simulink model "c00026M_harness"  (R2018a)
settings: Solver=ode3  StartTime=0.0  StopTime=10.0  RelTol=1e-3  EnableMultiTasking=on
undefined symbols (not defined in the file): b, DiscIntNeverNeededParam, J, K, L, PosMinimaW4, R, sigbuilder_block
(part 35 of 40)

== stateflow chart c00026M_harness/M063/Cyber/WL/Chart ==
  state Bajand_hasta_abajo
    entry: W = -1;
  state Bajando
    entry: W = -1;
  state Idle
    entry:W = 0;
  state Subiendo_hasta_arriba
    entry: W = 1;
  state Subiendo
    entry: W = 1;
  Subiendo -> Bajand_hasta_abajo [order 4] : [UI==4]
  Bajand_hasta_abajo -> Bajando [order 2] : [UI==3]
  Subiendo -> Bajando [order 3] : [UI==3]
  Bajando -> Bajand_hasta_abajo [order 2] : [UI==4]
  Idle -> Bajando [order 3] : [UI==3&&S>0]
  Subiendo_hasta_arriba -> Bajand_hasta_abajo [order 3] : [UI==4]
  Idle -> Bajand_hasta_abajo [order 4] : [UI==4&&S>0]
  Bajando -> Subiendo [order 3] : [UI==1]
  Subiendo_hasta_arriba -> Bajando [order 4] : [UI==3]
  Bajand_hasta_abajo -> Subiendo [order 4] : [UI==1]
  Bajand_hasta_abajo -> Idle [order 1] : [S<=0]
  Bajand_hasta_abajo -> Subiendo_hasta_arriba [order 3] : [UI==2]
  Bajando -> Idle [order 1] : [S<=0||UI==0]
  Bajando -> Subiendo_hasta_arriba [order 4] : [UI==2]
  (default) -> Idle
  Idle -> Subiendo_hasta_arriba [order 2] : [UI>2&&S<5]
  Idle -> Subiendo [order 1] : [UI == 1&&S<5]
  Subiendo -> Idle [order 1] : [S>=5||UI==0]
  Subiendo_hasta_arriba -> Idle [order 1] : [S >=5]
  Subiendo_hasta_arriba -> Subiendo [order 2] : [UI ==1]
  Subiendo -> Subiendo_hasta_arriba [order 2] : [UI==2]
  data: S input; UI input; W output double

== stateflow chart c00026M_harness/M063/Cyber/WL1/Chart1 ==
  state Bajand_hasta_abajo
    entry: W = -1;
  state Bajando
    entry: W = -1;
  state Idle
    entry:W = 0;
  state Subiendo_hasta_arriba
    entry: W = 1;
  state Subiendo
    entry: W = 1;
  Subiendo -> Bajand_hasta_abajo [order 4] : [UI==4]
  Bajand_hasta_abajo -> Bajando [order 2] : [UI==3]
  Subiendo -> Bajando [order 3] : [UI==3]
  Bajando -> Bajand_hasta_abajo [order 2] : [UI==4]
  Idle -> Bajando [order 3] : [UI==3&&S>0]
  Subiendo_hasta_arriba -> Bajand_hasta_abajo [order 3] : [UI==4]
  Idle -> Bajand_hasta_abajo [order 4] : [UI==4&&S>0]
  Bajando -> Subiendo [order 3] : [UI==1]
  Subiendo_hasta_arriba -> Bajando [order 4] : [UI==3]
  Bajand_hasta_abajo -> Subiendo [order 4] : [UI==1]
  Bajand_hasta_abajo -> Idle [order 1] : [S<=0]
  Bajand_hasta_abajo -> Subiendo_hasta_arriba [order 3] : [UI==2]
  Bajando -> Idle [order 1] : [S<=0||UI==0]
  Bajando -> Subiendo_hasta_arriba [order 4] : [UI==2]
  (default) -> Idle
  Idle -> Subiendo_hasta_arriba [order 2] : [UI==2&&S<5]
  Idle -> Subiendo [order 1] : [UI == 1&&S<5]
  Subiendo -> Idle [order 1] : [S>=5||UI==0]
  Subiendo_hasta_arriba -> Idle [order 1] : [S >=5]
  Subiendo_hasta_arriba -> Subiendo [order 2] : [UI ==1]
  Subiendo -> Subiendo_hasta_arriba [order 2] : [UI==2]
  data: S input; UI input; W output double

== stateflow chart c00026M_harness/M063/Cyber/WL3/Chart2 ==
  state Bajand_hasta_abajo
    entry: W = -1;
  state Bajando
    entry: W = -1;
  state Idle
    entry:W = 0;
  state Subiendo_hasta_arriba
    entry: W = 1;
  state Subiendo
    entry: W = 1;
  Subiendo -> Bajand_hasta_abajo [order 4] : [UI==4]
  Bajand_hasta_abajo -> Bajando [order 2] : [UI==3]
  Subiendo -> Bajando [order 3] : [UI==3]
  Bajando -> Bajand_hasta_abajo [order 2] : [UI==4]
  Idle -> Bajando [order 3] : [UI==3&&S>PosMinW4]
  Subiendo_hasta_arriba -> Bajand_hasta_abajo [order 3] : [UI==4]
  Idle -> Bajand_hasta_abajo [order 4] : [UI==4&&S>PosMinW4]
  Bajando -> Subiendo [order 3] : [UI==1]
  Subiendo_hasta_arriba -> Bajando [order 4] : [UI==3]
  Bajand_hasta_abajo -> Subiendo [order 4] : [UI==1]
  Bajand_hasta_abajo -> Idle [order 1] : [S<=PosMinW4]
  Bajand_hasta_abajo -> Subiendo_hasta_arriba [order 3] : [UI==2]
  Bajando -> Idle [order 1] : [S<=PosMinW4||UI==0]
  Bajando -> Subiendo_hasta_arriba [order 4] : [UI==2]
  (default) -> Idle
  Idle -> Subiendo_hasta_arriba [order 2] : [UI==2&&S<5]
  Idle -> Subiendo [order 1] : [UI == 1&&S<5]
  Subiendo -> Idle [order 1] : [S>=5||UI==0]
  Subiendo_hasta_arriba -> Idle [order 1] : [S >=5]
  Subiendo_hasta_arriba -> Subiendo [order 2] : [UI ==1]
  Subiendo -> Subiendo_hasta_arriba [order 2] : [UI==2]
  data: S input; UI input; W output double; PosMinW4 input

== stateflow chart c00026M_harness/M064/Cyber/WL/Chart ==
  state Bajand_hasta_abajo
    entry: W = -1;
  state Bajando
    entry: W = -1;
  state Idle
    entry:W = 0;
  state Subiendo_hasta_arriba
    entry: W = 1;
  state Subiendo
    entry: W = 1;
  Subiendo -> Bajand_hasta_abajo [order 4] : [UI==4]
  Bajand_hasta_abajo -> Bajando [order 2] : [UI==3]
  Subiendo -> Bajando [order 3] : [UI==3]
  Bajando -> Bajand_hasta_abajo [order 2] : [UI==4]
  Idle -> Bajando [order 3] : [UI==3&&S>0]
  Subiendo_hasta_arriba -> Bajand_hasta_abajo [order 3] : [UI==4]
  Idle -> Bajand_hasta_abajo [order 4] : [UI==4&&S>0]
  Bajando -> Subiendo [order 3] : [UI==1]
  Subiendo_hasta_arriba -> Bajando [order 4] : [UI==3]
  Bajand_hasta_abajo -> Subiendo [order 4] : [UI==1]
  Bajand_hasta_abajo -> Idle [order 1] : [S<=0]
  Bajand_hasta_abajo -> Subiendo_hasta_arriba [order 3] : [UI==2]
  Bajando -> Idle [order 1] : [S<=0||UI==0]
  Bajando -> Subiendo_hasta_arriba [order 4] : [UI==2]
  (default) -> Idle
  Idle -> Subiendo_hasta_arriba [order 2] : [UI==2&&S<5]
  Idle -> Subiendo [order 1] : [UI == 1&&S<5]
  Subiendo -> Idle [order 1] : [S>=5||UI==0]
  Subiendo_hasta_arriba -> Idle [order 1] : [S >=5]
  Subiendo_hasta_arriba -> Subiendo [order 2] : [UI ==1]
  Subiendo -> Subiendo_hasta_arriba [order 2] : [UI==2]
  data: S input; UI input; W output double

== stateflow chart c00026M_harness/M064/Cyber/WL1/Chart1 ==
  state Bajand_hasta_abajo
    entry: W = -1;
  state Bajando
    entry: W = -1;
  state Idle
    entry:W = 0;
  state Subiendo_hasta_arriba
    entry: W = 1;
  state Subiendo
    entry: W = 1;
  Subiendo -> Bajand_hasta_abajo [order 4] : [UI==4]
  Bajand_hasta_abajo -> Bajando [order 2] : [UI==3]
  Subiendo -> Bajando [order 3] : [UI==3]
  Bajando -> Bajand_hasta_abajo [order 2] : [UI==4]
  Idle -> Bajando [order 3] : [UI==3&&S>0]
  Subiendo_hasta_arriba -> Bajand_hasta_abajo [order 3] : [UI==4]
  Idle -> Bajand_hasta_abajo [order 4] : [UI==4&&S>0]
  Bajando -> Subiendo [order 3] : [UI==1]
  Subiendo_hasta_arriba -> Bajando [order 4] : [UI==3]
  Bajand_hasta_abajo -> Subiendo [order 4] : [UI==1]
  Bajand_hasta_abajo -> Idle [order 1] : [S<=0]
  Bajand_hasta_abajo -> Subiendo_hasta_arriba [order 3] : [UI==2]
  Bajando -> Idle [order 1] : [S<=0||UI==0]
  Bajando -> Subiendo_hasta_arriba [order 4] : [UI==2]
  (default) -> Idle
  Idle -> Subiendo_hasta_arriba [order 2] : [UI>2&&S<5]
  Idle -> Subiendo [order 1] : [UI == 1&&S<5]
  Subiendo -> Idle [order 1] : [S>=5||UI==0]
  Subiendo_hasta_arriba -> Idle [order 1] : [S >=5]
  Subiendo_hasta_arriba -> Subiendo [order 2] : [UI ==1]
  Subiendo -> Subiendo_hasta_arriba [order 2] : [UI==2]
  data: S input; UI input; W output double

== stateflow chart c00026M_harness/M064/Cyber/WL3/Chart2 ==
  state Bajand_hasta_abajo
    entry: W = -1;
  state Bajando
    entry: W = -1;
  state Idle
    entry:W = 0;
  state Subiendo_hasta_arriba
    entry: W = 1;
  state Subiendo
    entry: W = 1;
  Subiendo -> Bajand_hasta_abajo [order 4] : [UI==4]
  Bajand_hasta_abajo -> Bajando [order 2] : [UI==3]
  Subiendo -> Bajando [order 3] : [UI==3]
  Bajando -> Bajand_hasta_abajo [order 2] : [UI==4]
  Idle -> Bajando [order 3] : [UI==3&&S>PosMinW4]
  Subiendo_hasta_arriba -> Bajand_hasta_abajo [order 3] : [UI==4]
  Idle -> Bajand_hasta_abajo [order 4] : [UI==4&&S>PosMinW4]
  Bajando -> Subiendo [order 3] : [UI==1]
  Subiendo_hasta_arriba -> Bajando [order 4] : [UI==3]
  Bajand_hasta_abajo -> Subiendo [order 4] : [UI==1]
  Bajand_hasta_abajo -> Idle [order 1] : [S<=PosMinW4]
  Bajand_hasta_abajo -> Subiendo_hasta_arriba [order 3] : [UI==2]
  Bajando -> Idle [order 1] : [S<=PosMinW4||UI==0]
  Bajando -> Subiendo_hasta_arriba [order 4] : [UI==2]
  (default) -> Idle
  Idle -> Subiendo_hasta_arriba [order 2] : [UI==2&&S<5]
  Idle -> Subiendo [order 1] : [UI == 1&&S<5]
  Subiendo -> Idle [order 1] : [S>=5||UI==0]
  Subiendo_hasta_arriba -> Idle [order 1] : [S >=5]
  Subiendo_hasta_arriba -> Subiendo [order 2] : [UI ==1]
  Subiendo -> Subiendo_hasta_arriba [order 2] : [UI==2]
  data: S input; UI input; W output double; PosMinW4 input

== stateflow chart c00026M_harness/M066/Cyber/WL/Chart ==
  state Bajand_hasta_abajo
    entry: W = -1;
  state Bajando
    entry: W = -1;
  state Idle
    entry:W = 0;
  state Subiendo_hasta_arriba
    entry: W = 1;
  state Subiendo
    entry: W = 1;
  Subiendo -> Bajand_hasta_abajo [order 4] : [UI==4]
  Bajand_hasta_abajo -> Bajando [order 2] : [UI==3]
  Subiendo -> Bajando [order 3] : [UI==3]
  Bajando -> Bajand_hasta_abajo [order 2] : [UI==4]
  Idle -> Bajando [order 3] : [UI==3&&S>0]
  Subiendo_hasta_arriba -> Bajand_hasta_abajo [order 3] : [UI==4]
  Idle -> Bajand_hasta_abajo [order 4] : [UI==4&&S>0]
  Bajando -> Subiendo [order 3] : [UI==1]
  Subiendo_hasta_arriba -> Bajando [order 4] : [UI==3]
  Bajand_hasta_abajo -> Subiendo [order 4] : [UI==1]
  Bajand_hasta_abajo -> Idle [order 1] : [S<=0]
  Bajand_hasta_abajo -> Subiendo_hasta_arriba [order 3] : [UI==2]
  Bajando -> Idle [order 1] : [S<=0||UI==0]
  Bajando -> Subiendo_hasta_arriba [order 4] : [UI==2]
  (default) -> Idle
  Idle -> Subiendo_hasta_arriba [order 2] : [UI==2&&S<5]
  Idle -> Subiendo [order 1] : [UI == 1&&S<5]
  Subiendo -> Idle [order 1] : [S>=5||UI==0]
  Subiendo_hasta_arriba -> Idle [order 1] : [S >=5]
  Subiendo_hasta_arriba -> Subiendo [order 2] : [UI ==1]
  Subiendo -> Subiendo_hasta_arriba [order 2] : [UI==2]
  data: S input; UI input; W output double

== stateflow chart c00026M_harness/M066/Cyber/WL1/Chart1 ==
  state Bajand_hasta_abajo
    entry: W = -1;
  state Bajando
    entry: W = -1;
  state Idle
    entry:W = 0;
  state Subiendo_hasta_arriba
    entry: W = 1;
  state Subiendo
    entry: W = 1;
  Subiendo -> Bajand_hasta_abajo [order 4] : [UI==4]
  Bajand_hasta_abajo -> Bajando [order 2] : [UI==3]
  Subiendo -> Bajando [order 3] : [UI==3]
  Bajando -> Bajand_hasta_abajo [order 2] : [UI==4]
  Idle -> Bajando [order 3] : [UI==3&&S>0]
  Subiendo_hasta_arriba -> Bajand_hasta_abajo [order 3] : [UI==4]
  Idle -> Bajand_hasta_abajo [order 4] : [UI==4&&S>0]
  Bajando -> Subiendo [order 3] : [UI==1]
  Subiendo_hasta_arriba -> Bajando [order 4] : [UI==3]
  Bajand_hasta_abajo -> Subiendo [order 4] : [UI==1]
  Bajand_hasta_abajo -> Idle [order 1] : [S<=0]
  Bajand_hasta_abajo -> Subiendo_hasta_arriba [order 3] : [UI==2]
  Bajando -> Idle [order 1] : [S<=0||UI==0]
  Bajando -> Subiendo_hasta_arriba [order 4] : [UI==2]
  (default) -> Idle
  Idle -> Subiendo_hasta_arriba [order 2] : [UI==2&&S<5]
  Idle -> Subiendo [order 1] : [UI == 1&&S<5]
  Subiendo -> Idle [order 1] : [S>=5||UI==0]
  Subiendo_hasta_arriba -> Idle [order 1] : [S >=5]
  Subiendo_hasta_arriba -> Subiendo [order 2] : [UI ==1]
  Subiendo -> Subiendo_hasta_arriba [order 2] : [UI==2]
  data: S input; UI input; W output double

== stateflow chart c00026M_harness/M066/Cyber/WL3/Chart2 ==
  state Bajand_hasta_abajo
    entry: W = -1;
  state Bajando
    entry: W = -1;
  state Idle
    entry:W = 0;
  state Subiendo_hasta_arriba
    entry: W = 1;
  state Subiendo
    entry: W = 1;
  Subiendo -> Bajand_hasta_abajo [order 4] : [UI==4]
  Bajand_hasta_abajo -> Bajando [order 2] : [UI==3]
  Subiendo -> Bajando [order 3] : [UI==3]
  Bajando -> Bajand_hasta_abajo [order 2] : [UI==4]
  Idle -> Bajando [order 3] : [UI==3&&S>PosMinW4]
  Subiendo_hasta_arriba -> Bajand_hasta_abajo [order 3] : [UI==4]
  Idle -> Bajand_hasta_abajo [order 4] : [UI==4&&S>PosMinW4]
  Bajando -> Subiendo [order 3] : [UI==1]
  Subiendo_hasta_arriba -> Bajando [order 4] : [UI==3]
  Bajand_hasta_abajo -> Subiendo [order 4] : [UI==1]
  Bajand_hasta_abajo -> Idle [order 1] : [S<=PosMinW4]
  Bajand_hasta_abajo -> Subiendo_hasta_arriba [order 3] : [UI==2]
  Bajando -> Idle [order 1] : [S<=PosMinW4||UI==0]
  Bajando -> Subiendo_hasta_arriba [order 4] : [UI==2]
  (default) -> Idle
  Idle -> Subiendo_hasta_arriba [order 2] : [UI>2&&S<5]
  Idle -> Subiendo [order 1] : [UI == 1&&S<5]
  Subiendo -> Idle [order 1] : [S>=5||UI==0]
  Subiendo_hasta_arriba -> Idle [order 1] : [S >=5]
  Subiendo_hasta_arriba -> Subiendo [order 2] : [UI ==1]
  Subiendo -> Subiendo_hasta_arriba [order 2] : [UI==2]
  data: S input; UI input; W output double; PosMinW4 input

== stateflow chart c00026M_harness/M067/Cyber/WL/Chart ==
  state Bajand_hasta_abajo
    entry: W = -1;
  state Bajando
    entry: W = -1;
  state Idle
    entry:W = 0;
  state Subiendo_hasta_arriba
    entry: W = 1;
  state Subiendo
    entry: W = 1;
  Subiendo -> Bajand_hasta_abajo [order 4] : [UI==4]
  Bajand_hasta_abajo -> Bajando [order 2] : [UI==3]
  Subiendo -> Bajando [order 3] : [UI==3]
  Bajando -> Bajand_hasta_abajo [order 2] : [UI==4]
  Idle -> Bajando [order 3] : [UI==3&&S>0]
  Subiendo_hasta_arriba -> Bajand_hasta_abajo [order 3] : [UI==4]
  Idle -> Bajand_hasta_abajo [order 4] : [UI==4&&S>0]
  Bajando -> Subiendo [order 3] : [UI==1]
  Subiendo_hasta_arriba -> Bajando [order 4] : [UI==3]
  Bajand_hasta_abajo -> Subiendo [order 4] : [UI==1]
  Bajand_hasta_abajo -> Idle [order 1] : [S<=0]
  Bajand_hasta_abajo -> Subiendo_hasta_arriba [order 3] : [UI==2]
  Bajando -> Idle [order 1] : [S<=0||UI==0]
  Bajando -> Subiendo_hasta_arriba [order 4] : [UI==2]
  (default) -> Idle
  Idle -> Subiendo_hasta_arriba [order 2] : [UI==2&&S<5]
  Idle -> Subiendo [order 1] : [UI == 1&&S<5]
  Subiendo -> Idle [order 1] : [S>=5||UI==0]
  Subiendo_hasta_arriba -> Idle [order 1] : [S >=5]
  Subiendo_hasta_arriba -> Subiendo [order 2] : [UI ==1]
  Subiendo -> Subiendo_hasta_arriba [order 2] : [UI>2]
  data: S input; UI input; W output double

== stateflow chart c00026M_harness/M067/Cyber/WL1/Chart1 ==
  state Bajand_hasta_abajo
    entry: W = -1;
  state Bajando
    entry: W = -1;
  state Idle
    entry:W = 0;
  state Subiendo_hasta_arriba
    entry: W = 1;
  state Subiendo
    entry: W = 1;
  Subiendo -> Bajand_hasta_abajo [order 4] : [UI==4]
  Bajand_hasta_abajo -> Bajando [order 2] : [UI==3]
  Subiendo -> Bajando [order 3] : [UI==3]
  Bajando -> Bajand_hasta_abajo [order 2] : [UI==4]
  Idle -> Bajando [order 3] : [UI==3&&S>0]
  Subiendo_hasta_arriba -> Bajand_hasta_abajo [order 3] : [UI==4]
  Idle -> Bajand_hasta_abajo [order 4] : [UI==4&&S>0]
  Bajando -> Subiendo [order 3] : [UI==1]
  Subiendo_hasta_arriba -> Bajando [order 4] : [UI==3]
  Bajand_hasta_abajo -> Subiendo [order 4] : [UI==1]
  Bajand_hasta_abajo -> Idle [order 1] : [S<=0]
  Bajand_hasta_abajo -> Subiendo_hasta_arriba [order 3] : [UI==2]
  Bajando -> Idle [order 1] : [S<=0||UI==0]
  Bajando -> Subiendo_hasta_arriba [order 4] : [UI==2]
  (default) -> Idle
  Idle -> Subiendo_hasta_arriba [order 2] : [UI==2&&S<5]
  Idle -> Subiendo [order 1] : [UI == 1&&S<5]
  Subiendo -> Idle [order 1] : [S>=5||UI==0]
  Subiendo_hasta_arriba -> Idle [order 1] : [S >=5]
  Subiendo_hasta_arriba -> Subiendo [order 2] : [UI ==1]
  Subiendo -> Subiendo_hasta_arriba [order 2] : [UI==2]
  data: S input; UI input; W output double

== stateflow chart c00026M_harness/M067/Cyber/WL3/Chart2 ==
  state Bajand_hasta_abajo
    entry: W = -1;
  state Bajando
    entry: W = -1;
  state Idle
    entry:W = 0;
  state Subiendo_hasta_arriba
    entry: W = 1;
  state Subiendo
    entry: W = 1;
  Subiendo -> Bajand_hasta_abajo [order 4] : [UI==4]
  Bajand_hasta_abajo -> Bajando [order 2] : [UI==3]
  Subiendo -> Bajando [order 3] : [UI==3]
  Bajando -> Bajand_hasta_abajo [order 2] : [UI==4]
  Idle -> Bajando [order 3] : [UI==3&&S>PosMinW4]
  Subiendo_hasta_arriba -> Bajand_hasta_abajo [order 3] : [UI==4]
  Idle -> Bajand_hasta_abajo [order 4] : [UI==4&&S>PosMinW4]
  Bajando -> Subiendo [order 3] : [UI==1]
  Subiendo_hasta_arriba -> Bajando [order 4] : [UI==3]
  Bajand_hasta_abajo -> Subiendo [order 4] : [UI==1]
  Bajand_hasta_abajo -> Idle [order 1] : [S<=PosMinW4]
  Bajand_hasta_abajo -> Subiendo_hasta_arriba [order 3] : [UI==2]
  Bajando -> Idle [order 1] : [S<=PosMinW4||UI==0]
  Bajando -> Subiendo_hasta_arriba [order 4] : [UI==2]
  (default) -> Idle
  Idle -> Subiendo_hasta_arriba [order 2] : [UI==2&&S<5]
  Idle -> Subiendo [order 1] : [UI == 1&&S<5]
  Subiendo -> Idle [order 1] : [S>=5||UI==0]
  Subiendo_hasta_arriba -> Idle [order 1] : [S >=5]
  Subiendo_hasta_arriba -> Subiendo [order 2] : [UI ==1]
  Subiendo -> Subiendo_hasta_arriba [order 2] : [UI==2]
  data: S input; UI input; W output double; PosMinW4 input

== stateflow chart c00026M_harness/M068/Cyber/WL/Chart ==
  state Bajand_hasta_abajo
    entry: W = -1;
  state Bajando
    entry: W = -1;
  state Idle
    entry:W = 0;
  state Subiendo_hasta_arriba
    entry: W = 1;
  state Subiendo
    entry: W = 1;
  Subiendo -> Bajand_hasta_abajo [order 4] : [UI==4]
  Bajand_hasta_abajo -> Bajando [order 2] : [UI==3]
  Subiendo -> Bajando [order 3] : [UI==3]
  Bajando -> Bajand_hasta_abajo [order 2] : [UI==4]
  Idle -> Bajando [order 3] : [UI==3&&S>0]
  Subiendo_hasta_arriba -> Bajand_hasta_abajo [order 3] : [UI==4]
  Idle -> Bajand_hasta_abajo [order 4] : [UI==4&&S>0]
  Bajando -> Subiendo [order 3] : [UI==1]
  Subiendo_hasta_arriba -> Bajando [order 4] : [UI==3]
  Bajand_hasta_abajo -> Subiendo [order 4] : [UI==1]
  Bajand_hasta_abajo -> Idle [order 1] : [S<=0]
  Bajand_hasta_abajo -> Subiendo_hasta_arriba [order 3] : [UI==2]
  Bajando -> Idle [order 1] : [S<=0||UI==0]
  Bajando -> Subiendo_hasta_arriba [order 4] : [UI==2]
  (default) -> Idle
  Idle -> Subiendo_hasta_arriba [order 2] : [UI==2&&S<5]
  Idle -> Subiendo [order 1] : [UI == 1&&S<5]
  Subiendo -> Idle [order 1] : [S>=5||UI==0]
  Subiendo_hasta_arriba -> Idle [order 1] : [S >=5]
  Subiendo_hasta_arriba -> Subiendo [order 2] : [UI ==1]
  Subiendo -> Subiendo_hasta_arriba [order 2] : [UI==2]
  data: S input; UI input; W output double

== stateflow chart c00026M_harness/M068/Cyber/WL1/Chart1 ==
  state Bajand_hasta_abajo
    entry: W = -1;
  state Bajando
    entry: W = -1;
  state Idle
    entry:W = 0;
  state Subiendo_hasta_arriba
    entry: W = 1;
  state Subiendo
    entry: W = 1;
  Subiendo -> Bajand_hasta_abajo [order 4] : [UI==4]
  Bajand_hasta_abajo -> Bajando [order 2] : [UI==3]
  Subiendo -> Bajando [order 3] : [UI==3]
  Bajando -> Bajand_hasta_abajo [order 2] : [UI==4]
  Idle -> Bajando [order 3] : [UI==3&&S>0]
  Subiendo_hasta_arriba -> Bajand_hasta_abajo [order 3] : [UI==4]
  Idle -> Bajand_hasta_abajo [order 4] : [UI==4&&S>0]
  Bajando -> Subiendo [order 3] : [UI==1]
  Subiendo_hasta_arriba -> Bajando [order 4] : [UI==3]
  Bajand_hasta_abajo -> Subiendo [order 4] : [UI==1]
  Bajand_hasta_abajo -> Idle [order 1] : [S<=0]
  Bajand_hasta_abajo -> Subiendo_hasta_arriba [order 3] : [UI==2]
  Bajando -> Idle [order 1] : [S<=0||UI==0]
  Bajando -> Subiendo_hasta_arriba [order 4] : [UI==2]
  (default) -> Idle
  Idle -> Subiendo_hasta_arriba [order 2] : [UI==2&&S<5]
  Idle -> Subiendo [order 1] : [UI == 1&&S<5]
  Subiendo -> Idle [order 1] : [S>=5||UI==0]
  Subiendo_hasta_arriba -> Idle [order 1] : [S >=5]
  Subiendo_hasta_arriba -> Subiendo [order 2] : [UI ==1]
  Subiendo -> Subiendo_hasta_arriba [order 2] : [UI>2]
  data: S input; UI input; W output double

== stateflow chart c00026M_harness/M068/Cyber/WL3/Chart2 ==
  state Bajand_hasta_abajo
    entry: W = -1;
  state Bajando
    entry: W = -1;
  state Idle
    entry:W = 0;
  state Subiendo_hasta_arriba
    entry: W = 1;
  state Subiendo
    entry: W = 1;
  Subiendo -> Bajand_hasta_abajo [order 4] : [UI==4]
  Bajand_hasta_abajo -> Bajando [order 2] : [UI==3]
  Subiendo -> Bajando [order 3] : [UI==3]
  Bajando -> Bajand_hasta_abajo [order 2] : [UI==4]
  Idle -> Bajando [order 3] : [UI==3&&S>PosMinW4]
  Subiendo_hasta_arriba -> Bajand_hasta_abajo [order 3] : [UI==4]
  Idle -> Bajand_hasta_abajo [order 4] : [UI==4&&S>PosMinW4]
  Bajando -> Subiendo [order 3] : [UI==1]
  Subiendo_hasta_arriba -> Bajando [order 4] : [UI==3]
  Bajand_hasta_abajo -> Subiendo [order 4] : [UI==1]
  Bajand_hasta_abajo -> Idle [order 1] : [S<=PosMinW4]
  Bajand_hasta_abajo -> Subiendo_hasta_arriba [order 3] : [UI==2]
  Bajando -> Idle [order 1] : [S<=PosMinW4||UI==0]
  Bajando -> Subiendo_hasta_arriba [order 4] : [UI==2]
  (default) -> Idle
  Idle -> Subiendo_hasta_arriba [order 2] : [UI==2&&S<5]
  Idle -> Subiendo [order 1] : [UI == 1&&S<5]
  Subiendo -> Idle [order 1] : [S>=5||UI==0]
  Subiendo_hasta_arriba -> Idle [order 1] : [S >=5]
  Subiendo_hasta_arriba -> Subiendo [order 2] : [UI ==1]
  Subiendo -> Subiendo_hasta_arriba [order 2] : [UI==2]
  data: S input; UI input; W output double; PosMinW4 input

== stateflow chart c00026M_harness/M070/Cyber/WL/Chart ==
  state Bajand_hasta_abajo
    entry: W = -1;
  state Bajando
    entry: W = -1;
  state Idle
    entry:W = 0;
  state Subiendo_hasta_arriba
    entry: W = 1;
  state Subiendo
    entry: W = 1;
  Subiendo -> Bajand_hasta_abajo [order 4] : [UI==4]
  Bajand_hasta_abajo -> Bajando [order 2] : [UI==3]
  Subiendo -> Bajando [order 3] : [UI==3]
  Bajando -> Bajand_hasta_abajo [order 2] : [UI==4]
  Idle -> Bajando [order 3] : [UI==3&&S>0]
  Subiendo_hasta_arriba -> Bajand_hasta_abajo [order 3] : [UI==4]
  Idle -> Bajand_hasta_abajo [order 4] : [UI==4&&S>0]
  Bajando -> Subiendo [order 3] : [UI==1]
  Subiendo_hasta_arriba -> Bajando [order 4] : [UI==3]
  Bajand_hasta_abajo -> Subiendo [order 4] : [UI==1]
  Bajand_hasta_abajo -> Idle [order 1] : [S<=0]
  Bajand_hasta_abajo -> Subiendo_hasta_arriba [order 3] : [UI==2]
  Bajando -> Idle [order 1] : [S<=0||UI==0]
  Bajando -> Subiendo_hasta_arriba [order 4] : [UI==2]
  (default) -> Idle
  Idle -> Subiendo_hasta_arriba [order 2] : [UI==2&&S<5]
  Idle -> Subiendo [order 1] : [UI == 1&&S<5]
  Subiendo -> Idle [order 1] : [S>=5||UI==0]
  Subiendo_hasta_arriba -> Idle [order 1] : [S >=5]
  Subiendo_hasta_arriba -> Subiendo [order 2] : [UI ==1]
  Subiendo -> Subiendo_hasta_arriba [order 2] : [UI==2]
  data: S input; UI input; W output double

== stateflow chart c00026M_harness/M070/Cyber/WL1/Chart1 ==
  state Bajand_hasta_abajo
    entry: W = -1;
  state Bajando
    entry: W = -1;
  state Idle
    entry:W = 0;
  state Subiendo_hasta_arriba
    entry: W = 1;
  state Subiendo
    entry: W = 1;
  Subiendo -> Bajand_hasta_abajo [order 4] : [UI==4]
  Bajand_hasta_abajo -> Bajando [order 2] : [UI==3]
  Subiendo -> Bajando [order 3] : [UI==3]
  Bajando -> Bajand_hasta_abajo [order 2] : [UI==4]
  Idle -> Bajando [order 3] : [UI==3&&S>0]
  Subiendo_hasta_arriba -> Bajand_hasta_abajo [order 3] : [UI==4]
  Idle -> Bajand_hasta_abajo [order 4] : [UI==4&&S>0]
  Bajando -> Subiendo [order 3] : [UI==1]
  Subiendo_hasta_arriba -> Bajando [order 4] : [UI==3]
  Bajand_hasta_abajo -> Subiendo [order 4] : [UI==1]
  Bajand_hasta_abajo -> Idle [order 1] : [S<=0]
  Bajand_hasta_abajo -> Subiendo_hasta_arriba [order 3] : [UI==2]
  Bajando -> Idle [order 1] : [S<=0||UI==0]
  Bajando -> Subiendo_hasta_arriba [order 4] : [UI==2]
  (default) -> Idle
  Idle -> Subiendo_hasta_arriba [order 2] : [UI==2&&S<5]
  Idle -> Subiendo [order 1] : [UI == 1&&S<5]
  Subiendo -> Idle [order 1] : [S>=5||UI==0]
  Subiendo_hasta_arriba -> Idle [order 1] : [S >=5]
  Subiendo_hasta_arriba -> Subiendo [order 2] : [UI ==1]
  Subiendo -> Subiendo_hasta_arriba [order 2] : [UI==2]
  data: S input; UI input; W output double

== stateflow chart c00026M_harness/M070/Cyber/WL3/Chart2 ==
  state Bajand_hasta_abajo
    entry: W = -1;
  state Bajando
    entry: W = -1;
  state Idle
    entry:W = 0;
  state Subiendo_hasta_arriba
    entry: W = 1;
  state Subiendo
    entry: W = 1;
  Subiendo -> Bajand_hasta_abajo [order 4] : [UI==4]
  Bajand_hasta_abajo -> Bajando [order 2] : [UI==3]
  Subiendo -> Bajando [order 3] : [UI==3]
  Bajando -> Bajand_hasta_abajo [order 2] : [UI==4]
  Idle -> Bajando [order 3] : [UI==3&&S>PosMinW4]
  Subiendo_hasta_arriba -> Bajand_hasta_abajo [order 3] : [UI==4]
  Idle -> Bajand_hasta_abajo [order 4] : [UI==4&&S>PosMinW4]
  Bajando -> Subiendo [order 3] : [UI==1]
  Subiendo_hasta_arriba -> Bajando [order 4] : [UI==3]
  Bajand_hasta_abajo -> Subiendo [order 4] : [UI==1]
  Bajand_hasta_abajo -> Idle [order 1] : [S<=PosMinW4]
  Bajand_hasta_abajo -> Subiendo_hasta_arriba [order 3] : [UI==2]
  Bajando -> Idle [order 1] : [S<=PosMinW4||UI==0]
  Bajando -> Subiendo_hasta_arriba [order 4] : [UI==2]
  (default) -> Idle
  Idle -> Subiendo_hasta_arriba [order 2] : [UI==2&&S<5]
  Idle -> Subiendo [order 1] : [UI == 1&&S<5]
  Subiendo -> Idle [order 1] : [S>=5||UI==0]
  Subiendo_hasta_arriba -> Idle [order 1] : [S >=5]
  Subiendo_hasta_arriba -> Subiendo [order 2] : [UI ==1]
  Subiendo -> Subiendo_hasta_arriba [order 2] : [UI>2]
  data: S input; UI input; W output double; PosMinW4 input

== stateflow chart c00026M_harness/M071/Cyber/WL/Chart ==
  state Bajand_hasta_abajo
    entry: W = -1;
  state Bajando
    entry: W = -1;
  state Idle
    entry:W = 0;
  state Subiendo_hasta_arriba
    entry: W = 1;
  state Subiendo
    entry: W = 1;
  Subiendo -> Bajand_hasta_abajo [order 4] : [UI==4]
  Bajand_hasta_abajo -> Bajando [order 2] : [UI==3]
  Subiendo -> Bajando [order 3] : [UI==3]
  Bajando -> Bajand_hasta_abajo [order 2] : [UI==4]
  Idle -> Bajando [order 3] : [UI==3&&S>0]
  Subiendo_hasta_arriba -> Bajand_hasta_abajo [order 3] : [UI==4]
  Idle -> Bajand_hasta_abajo [order 4] : [UI==4&&S>0]
  Bajando -> Subiendo [order 3] : [UI==1]
  Subiendo_hasta_arriba -> Bajando [order 4] : [UI==3]
  Bajand_hasta_abajo -> Subiendo [order 4] : [UI==1]
  Bajand_hasta_abajo -> Idle [order 1] : [S<=0]
  Bajand_hasta_abajo -> Subiendo_hasta_arriba [order 3] : [UI==2]
  Bajando -> Idle [order 1] : [S<=0||UI==0]
  Bajando -> Subiendo_hasta_arriba [order 4] : [UI==2]
  (default) -> Idle
  Idle -> Subiendo_hasta_arriba [order 2] : [UI==2&&S<5]
  Idle -> Subiendo [order 1] : [UI == 1&&S<5]
  Subiendo -> Idle [order 1] : [S>=5||UI==0]
  Subiendo_hasta_arriba -> Idle [order 1] : [S >=5]
  Subiendo_hasta_arriba -> Subiendo [order 2] : [UI >1]
  Subiendo -> Subiendo_hasta_arriba [order 2] : [UI==2]
  data: S input; UI input; W output double

== stateflow chart c00026M_harness/M071/Cyber/WL1/Chart1 ==
  state Bajand_hasta_abajo
    entry: W = -1;
  state Bajando
    entry: W = -1;
  state Idle
    entry:W = 0;
  state Subiendo_hasta_arriba
    entry: W = 1;
  state Subiendo
    entry: W = 1;
  Subiendo -> Bajand_hasta_abajo [order 4] : [UI==4]
  Bajand_hasta_abajo -> Bajando [order 2] : [UI==3]
  Subiendo -> Bajando [order 3] : [UI==3]
  Bajando -> Bajand_hasta_abajo [order 2] : [UI==4]
  Idle -> Bajando [order 3] : [UI==3&&S>0]
  Subiendo_hasta_arriba -> Bajand_hasta_abajo [order 3] : [UI==4]
  Idle -> Bajand_hasta_abajo [order 4] : [UI==4&&S>0]
  Bajando -> Subiendo [order 3] : [UI==1]
  Subiendo_hasta_arriba -> Bajando [order 4] : [UI==3]
  Bajand_hasta_abajo -> Subiendo [order 4] : [UI==1]
  Bajand_hasta_abajo -> Idle [order 1] : [S<=0]
  Bajand_hasta_abajo -> Subiendo_hasta_arriba [order 3] : [UI==2]
  Bajando -> Idle [order 1] : [S<=0||UI==0]
  Bajando -> Subiendo_hasta_arriba [order 4] : [UI==2]
  (default) -> Idle
  Idle -> Subiendo_hasta_arriba [order 2] : [UI==2&&S<5]
  Idle -> Subiendo [order 1] : [UI == 1&&S<5]
  Subiendo -> Idle [order 1] : [S>=5||UI==0]
  Subiendo_hasta_arriba -> Idle [order 1] : [S >=5]
  Subiendo_hasta_arriba -> Subiendo [order 2] : [UI ==1]
  Subiendo -> Subiendo_hasta_arriba [order 2] : [UI==2]
  data: S input; UI input; W output double

== stateflow chart c00026M_harness/M071/Cyber/WL3/Chart2 ==
  state Bajand_hasta_abajo
    entry: W = -1;
  state Bajando
    entry: W = -1;
  state Idle
    entry:W = 0;
  state Subiendo_hasta_arriba
    entry: W = 1;
  state Subiendo
    entry: W = 1;
  Subiendo -> Bajand_hasta_abajo [order 4] : [UI==4]
  Bajand_hasta_abajo -> Bajando [order 2] : [UI==3]
  Subiendo -> Bajando [order 3] : [UI==3]
  Bajando -> Bajand_hasta_abajo [order 2] : [UI==4]
  Idle -> Bajando [order 3] : [UI==3&&S>PosMinW4]
  Subiendo_hasta_arriba -> Bajand_hasta_abajo [order 3] : [UI==4]
  Idle -> Bajand_hasta_abajo [order 4] : [UI==4&&S>PosMinW4]
  Bajando -> Subiendo [order 3] : [UI==1]
  Subiendo_hasta_arriba -> Bajando [order 4] : [UI==3]
  Bajand_hasta_abajo -> Subiendo [order 4] : [UI==1]
  Bajand_hasta_abajo -> Idle [order 1] : [S<=PosMinW4]
  Bajand_hasta_abajo -> Subiendo_hasta_arriba [order 3] : [UI==2]
  Bajando -> Idle [order 1] : [S<=PosMinW4||UI==0]
  Bajando -> Subiendo_hasta_arriba [order 4] : [UI==2]
  (default) -> Idle
  Idle -> Subiendo_hasta_arriba [order 2] : [UI==2&&S<5]
  Idle -> Subiendo [order 1] : [UI == 1&&S<5]
  Subiendo -> Idle [order 1] : [S>=5||UI==0]
  Subiendo_hasta_arriba -> Idle [order 1] : [S >=5]
  Subiendo_hasta_arriba -> Subiendo [order 2] : [UI ==1]
  Subiendo -> Subiendo_hasta_arriba [order 2] : [UI==2]
  data: S input; UI input; W output double; PosMinW4 input

== stateflow chart c00026M_harness/M072/Cyber/WL/Chart ==
  state Bajand_hasta_abajo
    entry: W = -1;
  state Bajando
    entry: W = -1;
  state Idle
    entry:W = 0;
  state Subiendo_hasta_arriba
    entry: W = 1;
  state Subiendo
    entry: W = 1;
  Subiendo -> Bajand_hasta_abajo [order 4] : [UI==4]
  Bajand_hasta_abajo -> Bajando [order 2] : [UI==3]
  Subiendo -> Bajando [order 3] : [UI==3]
  Bajando -> Bajand_hasta_abajo [order 2] : [UI==4]
  Idle -> Bajando [order 3] : [UI==3&&S>0]
  Subiendo_hasta_arriba -> Bajand_hasta_abajo [order 3] : [UI==4]
  Idle -> Bajand_hasta_abajo [order 4] : [UI==4&&S>0]
  Bajando -> Subiendo [order 3] : [UI==1]
  Subiendo_hasta_arriba -> Bajando [order 4] : [UI==3]
  Bajand_hasta_abajo -> Subiendo [order 4] : [UI==1]
  Bajand_hasta_abajo -> Idle [order 1] : [S<=0]
  Bajand_hasta_abajo -> Subiendo_hasta_arriba [order 3] : [UI==2]
  Bajando -> Idle [order 1] : [S<=0||UI==0]
  Bajando -> Subiendo_hasta_arriba [order 4] : [UI==2]
  (default) -> Idle
  Idle -> Subiendo_hasta_arriba [order 2] : [UI==2&&S<5]
  Idle -> Subiendo [order 1] : [UI == 1&&S<5]
  Subiendo -> Idle [order 1] : [S>=5||UI==0]
  Subiendo_hasta_arriba -> Idle [order 1] : [S >=5]
  Subiendo_hasta_arriba -> Subiendo [order 2] : [UI ==1]
  Subiendo -> Subiendo_hasta_arriba [order 2] : [UI==2]
  data: S input; UI input; W output double

== stateflow chart c00026M_harness/M072/Cyber/WL1/Chart1 ==
  state Bajand_hasta_abajo
    entry: W = -1;
  state Bajando
    entry: W = -1;
  state Idle
    entry:W = 0;
  state Subiendo_hasta_arriba
    entry: W = 1;
  state Subiendo
    entry: W = 1;
  Subiendo -> Bajand_hasta_abajo [order 4] : [UI==4]
  Bajand_hasta_abajo -> Bajando [order 2] : [UI==3]
  Subiendo -> Bajando [order 3] : [UI==3]
  Bajando -> Bajand_hasta_abajo [order 2] : [UI==4]
  Idle -> Bajando [order 3] : [UI==3&&S>0]
  Subiendo_hasta_arriba -> Bajand_hasta_abajo [order 3] : [UI==4]
  Idle -> Bajand_hasta_abajo [order 4] : [UI==4&&S>0]
  Bajando -> Subiendo [order 3] : [UI==1]
  Subiendo_hasta_arriba -> Bajando [order 4] : [UI==3]
  Bajand_hasta_abajo -> Subiendo [order 4] : [UI==1]
  Bajand_hasta_abajo -> Idle [order 1] : [S<=0]
  Bajand_hasta_abajo -> Subiendo_hasta_arriba [order 3] : [UI==2]
  Bajando -> Idle [order 1] : [S<=0||UI==0]
  Bajando -> Subiendo_hasta_arriba [order 4] : [UI==2]
  (default) -> Idle
  Idle -> Subiendo_hasta_arriba [order 2] : [UI==2&&S<5]
  Idle -> Subiendo [order 1] : [UI == 1&&S<5]
  Subiendo -> Idle [order 1] : [S>=5||UI==0]
  Subiendo_hasta_arriba -> Idle [order 1] : [S >=5]
  Subiendo_hasta_arriba -> Subiendo [order 2] : [UI >1]
  Subiendo -> Subiendo_hasta_arriba [order 2] : [UI==2]
  data: S input; UI input; W output double

== stateflow chart c00026M_harness/M072/Cyber/WL3/Chart2 ==
  state Bajand_hasta_abajo
    entry: W = -1;
  state Bajando
    entry: W = -1;
  state Idle
    entry:W = 0;
  state Subiendo_hasta_arriba
    entry: W = 1;
  state Subiendo
    entry: W = 1;
  Subiendo -> Bajand_hasta_abajo [order 4] : [UI==4]
  Bajand_hasta_abajo -> Bajando [order 2] : [UI==3]
  Subiendo -> Bajando [order 3] : [UI==3]
  Bajando -> Bajand_hasta_abajo [order 2] : [UI==4]
  Idle -> Bajando [order 3] : [UI==3&&S>PosMinW4]
  Subiendo_hasta_arriba -> Bajand_hasta_abajo [order 3] : [UI==4]
  Idle -> Bajand_hasta_abajo [order 4] : [UI==4&&S>PosMinW4]
  Bajando -> Subiendo [order 3] : [UI==1]
  Subiendo_hasta_arriba -> Bajando [order 4] : [UI==3]
  Bajand_hasta_abajo -> Subiendo [order 4] : [UI==1]
  Bajand_hasta_abajo -> Idle [order 1] : [S<=PosMinW4]
  Bajand_hasta_abajo -> Subiendo_hasta_arriba [order 3] : [UI==2]
  Bajando -> Idle [order 1] : [S<=PosMinW4||UI==0]
  Bajando -> Subiendo_hasta_arriba [order 4] : [UI==2]
  (default) -> Idle
  Idle -> Subiendo_hasta_arriba [order 2] : [UI==2&&S<5]
  Idle -> Subiendo [order 1] : [UI == 1&&S<5]
  Subiendo -> Idle [order 1] : [S>=5||UI==0]
  Subiendo_hasta_arriba -> Idle [order 1] : [S >=5]
  Subiendo_hasta_arriba -> Subiendo [order 2] : [UI ==1]
  Subiendo -> Subiendo_hasta_arriba [order 2] : [UI==2]
  data: S input; UI input; W output double; PosMinW4 input

== stateflow chart c00026M_harness/M074/Cyber/WL/Chart ==
  state Bajand_hasta_abajo
    entry: W = -1;
  state Bajando
    entry: W = -1;
  state Idle
    entry:W = 0;
  state Subiendo_hasta_arriba
    entry: W = 1;
  state Subiendo
    entry: W = 1;
  Subiendo -> Bajand_hasta_abajo [order 4] : [UI==4]
  Bajand_hasta_abajo -> Bajando [order 2] : [UI==3]
  Subiendo -> Bajando [order 3] : [UI==3]
  Bajando -> Bajand_hasta_abajo [order 2] : [UI==4]
  Idle -> Bajando [order 3] : [UI==3&&S>0]
  Subiendo_hasta_arriba -> Bajand_hasta_abajo [order 3] : [UI==4]
  Idle -> Bajand_hasta_abajo [order 4] : [UI==4&&S>0]
  Bajando -> Subiendo [order 3] : [UI==1]
  Subiendo_hasta_arriba -> Bajando [order 4] : [UI==3]
  Bajand_hasta_abajo -> Subiendo [order 4] : [UI==1]
  Bajand_hasta_abajo -> Idle [order 1] : [S<=0]
  Bajand_hasta_abajo -> Subiendo_hasta_arriba [order 3] : [UI==2]
  Bajando -> Idle [order 1] : [S<=0||UI==0]
  Bajando -> Subiendo_hasta_arriba [order 4] : [UI==2]
  (default) -> Idle
  Idle -> Subiendo_hasta_arriba [order 2] : [UI==2&&S<5]
  Idle -> Subiendo [order 1] : [UI == 1&&S<5]
  Subiendo -> Idle [order 1] : [S>=5||UI==0]
  Subiendo_hasta_arriba -> Idle [order 1] : [S >=5]
  Subiendo_hasta_arriba -> Subiendo [order 2] : [UI ==1]
  Subiendo -> Subiendo_hasta_arriba [order 2] : [UI==2]
  data: S input; UI input; W output double

== stateflow chart c00026M_harness/M074/Cyber/WL1/Chart1 ==
  state Bajand_hasta_abajo
    entry: W = -1;
  state Bajando
    entry: W = -1;
  state Idle
    entry:W = 0;
  state Subiendo_hasta_arriba
    entry: W = 1;
  state Subiendo
    entry: W = 1;
  Subiendo -> Bajand_hasta_abajo [order 4] : [UI==4]
  Bajand_hasta_abajo -> Bajando [order 2] : [UI==3]
  Subiendo -> Bajando [order 3] : [UI==3]
  Bajando -> Bajand_hasta_abajo [order 2] : [UI==4]
  Idle -> Bajando [order 3] : [UI==3&&S>0]
  Subiendo_hasta_arriba -> Bajand_hasta_abajo [order 3] : [UI==4]
  Idle -> Bajand_hasta_abajo [order 4] : [UI==4&&S>0]
  Bajando -> Subiendo [order 3] : [UI==1]
  Subiendo_hasta_arriba -> Bajando [order 4] : [UI==3]
  Bajand_hasta_abajo -> Subiendo [order 4] : [UI==1]
  Bajand_hasta_abajo -> Idle [order 1] : [S<=0]
  Bajand_hasta_abajo -> Subiendo_hasta_arriba [order 3] : [UI==2]
  Bajando -> Idle [order 1] : [S<=0||UI==0]
  Bajando -> Subiendo_hasta_arriba [order 4] : [UI==2]
  (default) -> Idle
  Idle -> Subiendo_hasta_arriba [order 2] : [UI==2&&S<5]
  Idle -> Subiendo [order 1] : [UI == 1&&S<5]
  Subiendo -> Idle [order 1] : [S>=5||UI==0]
  Subiendo_hasta_arriba -> Idle [order 1] : [S >=5]
  Subiendo_hasta_arriba -> Subiendo [order 2] : [UI ==1]
  Subiendo -> Subiendo_hasta_arriba [order 2] : [UI==2]
  data: S input; UI input; W output double

== stateflow chart c00026M_harness/M074/Cyber/WL3/Chart2 ==
  state Bajand_hasta_abajo
    entry: W = -1;
  state Bajando
    entry: W = -1;
  state Idle
    entry:W = 0;
  state Subiendo_hasta_arriba
    entry: W = 1;
  state Subiendo
    entry: W = 1;
  Subiendo -> Bajand_hasta_abajo [order 4] : [UI==4]
  Bajand_hasta_abajo -> Bajando [order 2] : [UI==3]
  Subiendo -> Bajando [order 3] : [UI==3]
  Bajando -> Bajand_hasta_abajo [order 2] : [UI==4]
  Idle -> Bajando [order 3] : [UI==3&&S>PosMinW4]
  Subiendo_hasta_arriba -> Bajand_hasta_abajo [order 3] : [UI==4]
  Idle -> Bajand_hasta_abajo [order 4] : [UI==4&&S>PosMinW4]
  Bajando -> Subiendo [order 3] : [UI==1]
  Subiendo_hasta_arriba -> Bajando [order 4] : [UI==3]
  Bajand_hasta_abajo -> Subiendo [order 4] : [UI==1]
  Bajand_hasta_abajo -> Idle [order 1] : [S<=PosMinW4]
  Bajand_hasta_abajo -> Subiendo_hasta_arriba [order 3] : [UI==2]
  Bajando -> Idle [order 1] : [S<=PosMinW4||UI==0]
  Bajando -> Subiendo_hasta_arriba [order 4] : [UI==2]
  (default) -> Idle
  Idle -> Subiendo_hasta_arriba [order 2] : [UI==2&&S<5]
  Idle -> Subiendo [order 1] : [UI == 1&&S<5]
  Subiendo -> Idle [order 1] : [S>=5||UI==0]
  Subiendo_hasta_arriba -> Idle [order 1] : [S >=5]
  Subiendo_hasta_arriba -> Subiendo [order 2] : [UI >1]
  Subiendo -> Subiendo_hasta_arriba [order 2] : [UI==2]
  data: S input; UI input; W output double; PosMinW4 input

== stateflow chart c00026M_harness/M075/Cyber/WL/Chart ==
  state Bajand_hasta_abajo
    entry: W = -1;
  state Bajando
    entry: W = -1;
  state Idle
    entry:W = 0;
  state Subiendo_hasta_arriba
    entry: W = 1;
  state Subiendo
    entry: W = 1;
  Subiendo -> Bajand_hasta_abajo [order 4] : [UI==4]
  Bajand_hasta_abajo -> Bajando [order 2] : [UI==3]
  Subiendo -> Bajando [order 3] : [UI==3]
  Bajando -> Bajand_hasta_abajo [order 2] : [UI==4]
  Idle -> Bajando [order 3] : [UI==3&&S>0]
  Subiendo_hasta_arriba -> Bajand_hasta_abajo [order 3] : [UI==4]
  Idle -> Bajand_hasta_abajo [order 4] : [UI==4&&S>0]
  Bajando -> Subiendo [order 3] : [UI>1]
  Subiendo_hasta_arriba -> Bajando [order 4] : [UI==3]
  Bajand_hasta_abajo -> Subiendo [order 4] : [UI==1]
  Bajand_hasta_abajo -> Idle [order 1] : [S<=0]
  Bajand_hasta_abajo -> Subiendo_hasta_arriba [order 3] : [UI==2]
  Bajando -> Idle [order 1] : [S<=0||UI==0]
  Bajando -> Subiendo_hasta_arriba [order 4] : [UI==2]
  (default) -> Idle
  Idle -> Subiendo_hasta_arriba [order 2] : [UI==2&&S<5]
  Idle -> Subiendo [order 1] : [UI == 1&&S<5]
  Subiendo -> Idle [order 1] : [S>=5||UI==0]
  Subiendo_hasta_arriba -> Idle [order 1] : [S >=5]
  Subiendo_hasta_arriba -> Subiendo [order 2] : [UI ==1]
  Subiendo -> Subiendo_hasta_arriba [order 2] : [UI==2]
  data: S input; UI input; W output double

== stateflow chart c00026M_harness/M075/Cyber/WL1/Chart1 ==
  state Bajand_hasta_abajo
    entry: W = -1;
  state Bajando
    entry: W = -1;
  state Idle
    entry:W = 0;
  state Subiendo_hasta_arriba
    entry: W = 1;
  state Subiendo
    entry: W = 1;
  Subiendo -> Bajand_hasta_abajo [order 4] : [UI==4]
  Bajand_hasta_abajo -> Bajando [order 2] : [UI==3]
  Subiendo -> Bajando [order 3] : [UI==3]
  Bajando -> Bajand_hasta_abajo [order 2] : [UI==4]
  Idle -> Bajando [order 3] : [UI==3&&S>0]
  Subiendo_hasta_arriba -> Bajand_hasta_abajo [order 3] : [UI==4]
  Idle -> Bajand_hasta_abajo [order 4] : [UI==4&&S>0]
  Bajando -> Subiendo [order 3] : [UI==1]
  Subiendo_hasta_arriba -> Bajando [order 4] : [UI==3]
  Bajand_hasta_abajo -> Subiendo [order 4] : [UI==1]
  Bajand_hasta_abajo -> Idle [order 1] : [S<=0]
  Bajand_hasta_abajo -> Subiendo_hasta_arriba [order 3] : [UI==2]
  Bajando -> Idle [order 1] : [S<=0||UI==0]
  Bajando -> Subiendo_hasta_arriba [order 4] : [UI==2]
  (default) -> Idle
  Idle -> Subiendo_hasta_arriba [order 2] : [UI==2&&S<5]
  Idle -> Subiendo [order 1] : [UI == 1&&S<5]
  Subiendo -> Idle [order 1] : [S>=5||UI==0]
  Subiendo_hasta_arriba -> Idle [order 1] : [S >=5]
  Subiendo_hasta_arriba -> Subiendo [order 2] : [UI ==1]
  Subiendo -> Subiendo_hasta_arriba [order 2] : [UI==2]
  data: S input; UI input; W output double

== stateflow chart c00026M_harness/M075/Cyber/WL3/Chart2 ==
  state Bajand_hasta_abajo
    entry: W = -1;
  state Bajando
    entry: W = -1;
  state Idle
    entry:W = 0;
  state Subiendo_hasta_arriba
    entry: W = 1;
  state Subiendo
    entry: W = 1;
  Subiendo -> Bajand_hasta_abajo [order 4] : [UI==4]
  Bajand_hasta_abajo -> Bajando [order 2] : [UI==3]
  Subiendo -> Bajando [order 3] : [UI==3]
  Bajando -> Bajand_hasta_abajo [order 2] : [UI==4]
  Idle -> Bajando [order 3] : [UI==3&&S>PosMinW4]
  Subiendo_hasta_arriba -> Bajand_hasta_abajo [order 3] : [UI==4]
  Idle -> Bajand_hasta_abajo [order 4] : [UI==4&&S>PosMinW4]
  Bajando -> Subiendo [order 3] : [UI==1]
  Subiendo_hasta_arriba -> Bajando [order 4] : [UI==3]
  Bajand_hasta_abajo -> Subiendo [order 4] : [UI==1]
  Bajand_hasta_abajo -> Idle [order 1] : [S<=PosMinW4]
  Bajand_hasta_abajo -> Subiendo_hasta_arriba [order 3] : [UI==2]
  Bajando -> Idle [order 1] : [S<=PosMinW4||UI==0]
  Bajando -> Subiendo_hasta_arriba [order 4] : [UI==2]
  (default) -> Idle
  Idle -> Subiendo_hasta_arriba [order 2] : [UI==2&&S<5]
  Idle -> Subiendo [order 1] : [UI == 1&&S<5]
  Subiendo -> Idle [order 1] : [S>=5||UI==0]
  Subiendo_hasta_arriba -> Idle [order 1] : [S >=5]
  Subiendo_hasta_arriba -> Subiendo [order 2] : [UI ==1]
  Subiendo -> Subiendo_hasta_arriba [order 2] : [UI==2]
  data: S input; UI input; W output double; PosMinW4 input

== stateflow chart c00026M_harness/M076/Cyber/WL/Chart ==
  state Bajand_hasta_abajo
    entry: W = -1;
  state Bajando
    entry: W = -1;
  state Idle
    entry:W = 0;
  state Subiendo_hasta_arriba
    entry: W = 1;
  state Subiendo
    entry: W = 1;
  Subiendo -> Bajand_hasta_abajo [order 4] : [UI==4]
  Bajand_hasta_abajo -> Bajando [order 2] : [UI==3]
  Subiendo -> Bajando [order 3] : [UI==3]
  Bajando -> Bajand_hasta_abajo [order 2] : [UI==4]
  Idle -> Bajando [order 3] : [UI==3&&S>0]
  Subiendo_hasta_arriba -> Bajand_hasta_abajo [order 3] : [UI==4]
  Idle -> Bajand_hasta_abajo [order 4] : [UI==4&&S>0]
  Bajando -> Subiendo [order 3] : [UI==1]
  Subiendo_hasta_arriba -> Bajando [order 4] : [UI==3]
  Bajand_hasta_abajo -> Subiendo [order 4] : [UI==1]
  Bajand_hasta_abajo -> Idle [order 1] : [S<=0]
  Bajand_hasta_abajo -> Subiendo_hasta_arriba [order 3] : [UI==2]
  Bajando -> Idle [order 1] : [S<=0||UI==0]
  Bajando -> Subiendo_hasta_arriba [order 4] : [UI==2]
  (default) -> Idle
  Idle -> Subiendo_hasta_arriba [order 2] : [UI==2&&S<5]
  Idle -> Subiendo [order 1] : [UI == 1&&S<5]
  Subiendo -> Idle [order 1] : [S>=5||UI==0]
  Subiendo_hasta_arriba -> Idle [order 1] : [S >=5]
  Subiendo_hasta_arriba -> Subiendo [order 2] : [UI ==1]
  Subiendo -> Subiendo_hasta_arriba [order 2] : [UI==2]
  data: S input; UI input; W output double

== stateflow chart c00026M_harness/M076/Cyber/WL1/Chart1 ==
  state Bajand_hasta_abajo
    entry: W = -1;
  state Bajando
    entry: W = -1;
  state Idle
    entry:W = 0;
  state Subiendo_hasta_arriba
    entry: W = 1;
  state Subiendo
    entry: W = 1;
  Subiendo -> Bajand_hasta_abajo [order 4] : [UI==4]
  Bajand_hasta_abajo -> Bajando [order 2] : [UI==3]
  Subiendo -> Bajando [order 3] : [UI==3]
  Bajando -> Bajand_hasta_abajo [order 2] : [UI==4]
  Idle -> Bajando [order 3] : [UI==3&&S>0]
  Subiendo_hasta_arriba -> Bajand_hasta_abajo [order 3] : [UI==4]
  Idle -> Bajand_hasta_abajo [order 4] : [UI==4&&S>0]
  Bajando -> Subiendo [order 3] : [UI>1]
  Subiendo_hasta_arriba -> Bajando [order 4] : [UI==3]
  Bajand_hasta_abajo -> Subiendo [order 4] : [UI==1]
  Bajand_hasta_abajo -> Idle [order 1] : [S<=0]
  Bajand_hasta_abajo -> Subiendo_hasta_arriba [order 3] : [UI==2]
  Bajando -> Idle [order 1] : [S<=0||UI==0]
  Bajando -> Subiendo_hasta_arriba [order 4] : [UI==2]
  (default) -> Idle
  Idle -> Subiendo_hasta_arriba [order 2] : [UI==2&&S<5]
  Idle -> Subiendo [order 1] : [UI == 1&&S<5]
  Subiendo -> Idle [order 1] : [S>=5||UI==0]
  Subiendo_hasta_arriba -> Idle [order 1] : [S >=5]
  Subiendo_hasta_arriba -> Subiendo [order 2] : [UI ==1]
  Subiendo -> Subiendo_hasta_arriba [order 2] : [UI==2]
  data: S input; UI input; W output double

== stateflow chart c00026M_harness/M076/Cyber/WL3/Chart2 ==
  state Bajand_hasta_abajo
    entry: W = -1;
  state Bajando
    entry: W = -1;
  state Idle
    entry:W = 0;
  state Subiendo_hasta_arriba
    entry: W = 1;
  state Subiendo
    entry: W = 1;
  Subiendo -> Bajand_hasta_abajo [order 4] : [UI==4]
  Bajand_hasta_abajo -> Bajando [order 2] : [UI==3]
  Subiendo -> Bajando [order 3] : [UI==3]
  Bajando -> Bajand_hasta_abajo [order 2] : [UI==4]
  Idle -> Bajando [order 3] : [UI==3&&S>PosMinW4]
  Subiendo_hasta_arriba -> Bajand_hasta_abajo [order 3] : [UI==4]
  Idle -> Bajand_hasta_abajo [order 4] : [UI==4&&S>PosMinW4]
  Bajando -> Subiendo [order 3] : [UI==1]
  Subiendo_hasta_arriba -> Bajando [order 4] : [UI==3]
  Bajand_hasta_abajo -> Subiendo [order 4] : [UI==1]
  Bajand_hasta_abajo -> Idle [order 1] : [S<=PosMinW4]
  Bajand_hasta_abajo -> Subiendo_hasta_arriba [order 3] : [UI==2]
  Bajando -> Idle [order 1] : [S<=PosMinW4||UI==0]
  Bajando -> Subiendo_hasta_arriba [order 4] : [UI==2]
  (default) -> Idle
  Idle -> Subiendo_hasta_arriba [order 2] : [UI==2&&S<5]
  Idle -> Subiendo [order 1] : [UI == 1&&S<5]
  Subiendo -> Idle [order 1] : [S>=5||UI==0]
  Subiendo_hasta_arriba -> Idle [order 1] : [S >=5]
  Subiendo_hasta_arriba -> Subiendo [order 2] : [UI ==1]
  Subiendo -> Subiendo_hasta_arriba [order 2] : [UI==2]
  data: S input; UI input; W output double; PosMinW4 input

== stateflow chart c00026M_harness/M078/Cyber/WL/Chart ==
  state Bajand_hasta_abajo
    entry: W = -1;
  state Bajando
    entry: W = -1;
  state Idle
    entry:W = 0;
  state Subiendo_hasta_arriba
    entry: W = 1;
  state Subiendo
    entry: W = 1;
  Subiendo -> Bajand_hasta_abajo [order 4] : [UI==4]
  Bajand_hasta_abajo -> Bajando [order 2] : [UI==3]
  Subiendo -> Bajando [order 3] : [UI==3]
  Bajando -> Bajand_hasta_abajo [order 2] : [UI==4]
  Idle -> Bajando [order 3] : [UI==3&&S>0]
  Subiendo_hasta_arriba -> Bajand_hasta_abajo [order 3] : [UI==4]
  Idle -> Bajand_hasta_abajo [order 4] : [UI==4&&S>0]
  Bajando -> Subiendo [order 3] : [UI==1]
  Subiendo_hasta_arriba -> Bajando [order 4] : [UI==3]
  Bajand_hasta_abajo -> Subiendo [order 4] : [UI==1]
  Bajand_hasta_abajo -> Idle [order 1] : [S<=0]
  Bajand_hasta_abajo -> Subiendo_hasta_arriba [order 3] : [UI==2]
  Bajando -> Idle [order 1] : [S<=0||UI==0]
  Bajando -> Subiendo_hasta_arriba [order 4] : [UI==2]
  (default) -> Idle
  Idle -> Subiendo_hasta_arriba [order 2] : [UI==2&&S<5]
  Idle -> Subiendo [order 1] : [UI == 1&&S<5]
  Subiendo -> Idle [order 1] : [S>=5||UI==0]
  Subiendo_hasta_arriba -> Idle [order 1] : [S >=5]
  Subiendo_hasta_arriba -> Subiendo [order 2] : [UI ==1]
  Subiendo -> Subiendo_hasta_arriba [order 2] : [UI==2]
  data: S input; UI input; W output double

== stateflow chart c00026M_harness/M078/Cyber/WL1/Chart1 ==
  state Bajand_hasta_abajo
    entry: W = -1;
  state Bajando
    entry: W = -1;
  state Idle
    entry:W = 0;
  state Subiendo_hasta_arriba
    entry: W = 1;
  state Subiendo
    entry: W = 1;
  Subiendo -> Bajand_hasta_abajo [order 4] : [UI==4]
  Bajand_hasta_abajo -> Bajando [order 2] : [UI==3]
  Subiendo -> Bajando [order 3] : [UI==3]
  Bajando -> Bajand_hasta_abajo [order 2] : [UI==4]
  Idle -> Bajando [order 3] : [UI==3&&S>0]
  Subiendo_hasta_arriba -> Bajand_hasta_abajo [order 3] : [UI==4]
  Idle -> Bajand_hasta_abajo [order 4] : [UI==4&&S>0]
  Bajando -> Subiendo [order 3] : [UI==1]
  Subiendo_hasta_arriba -> Bajando [order 4] : [UI==3]
  Bajand_hasta_abajo -> Subiendo [order 4] : [UI==1]
  Bajand_hasta_abajo -> Idle [order 1] : [S<=0]
  Bajand_hasta_abajo -> Subiendo_hasta_arriba [order 3] : [UI==2]
  Bajando -> Idle [order 1] : [S<=0||UI==0]
  Bajando -> Subiendo_hasta_arriba [order 4] : [UI==2]
  (default) -> Idle
  Idle -> Subiendo_hasta_arriba [order 2] : [UI==2&&S<5]
  Idle -> Subiendo [order 1] : [UI == 1&&S<5]
  Subiendo -> Idle [order 1] : [S>=5||UI==0]
  Subiendo_hasta_arriba -> Idle [order 1] : [S >=5]
  Subiendo_hasta_arriba -> Subiendo [order 2] : [UI ==1]
  Subiendo -> Subiendo_hasta_arriba [order 2] : [UI==2]
  data: S input; UI input; W output double

== stateflow chart c00026M_harness/M078/Cyber/WL3/Chart2 ==
  state Bajand_hasta_abajo
    entry: W = -1;
  state Bajando
    entry: W = -1;
  state Idle
    entry:W = 0;
  state Subiendo_hasta_arriba
    entry: W = 1;
  state Subiendo
    entry: W = 1;
  Subiendo -> Bajand_hasta_abajo [order 4] : [UI==4]
  Bajand_hasta_abajo -> Bajando [order 2] : [UI==3]
  Subiendo -> Bajando [order 3] : [UI==3]
  Bajando -> Bajand_hasta_abajo [order 2] : [UI==4]
  Idle -> Bajando [order 3] : [UI==3&&S>PosMinW4]
  Subiendo_hasta_arriba -> Bajand_hasta_abajo [order 3] : [UI==4]
  Idle -> Bajand_hasta_abajo [order 4] : [UI==4&&S>PosMinW4]
  Bajando -> Subiendo [order 3] : [UI>1]
  Subiendo_hasta_arriba -> Bajando [order 4] : [UI==3]
  Bajand_hasta_abajo -> Subiendo [order 4] : [UI==1]
  Bajand_hasta_abajo -> Idle [order 1] : [S<=PosMinW4]
  Bajand_hasta_abajo -> Subiendo_hasta_arriba [order 3] : [UI==2]
  Bajando -> Idle [order 1] : [S<=PosMinW4||UI==0]
  Bajando -> Subiendo_hasta_arriba [order 4] : [UI==2]
  (default) -> Idle
  Idle -> Subiendo_hasta_arriba [order 2] : [UI==2&&S<5]
  Idle -> Subiendo [order 1] : [UI == 1&&S<5]
  Subiendo -> Idle [order 1] : [S>=5||UI==0]
  Subiendo_hasta_arriba -> Idle [order 1] : [S >=5]
  Subiendo_hasta_arriba -> Subiendo [order 2] : [UI ==1]
  Subiendo -> Subiendo_hasta_arriba [order 2] : [UI==2]
  data: S input; UI input; W output double; PosMinW4 input

== stateflow chart c00026M_harness/M079/Cyber/WL/Chart ==
  state Bajand_hasta_abajo
    entry: W = -1;
  state Bajando
    entry: W = -1;
  state Idle
    entry:W = 0;
  state Subiendo_hasta_arriba
    entry: W = 1;
  state Subiendo
    entry: W = 1;
  Subiendo -> Bajand_hasta_abajo [order 4] : [UI==4]
  Bajand_hasta_abajo -> Bajando [order 2] : [UI==3]
  Subiendo -> Bajando [order 3] : [UI==3]
  Bajando -> Bajand_hasta_abajo [order 2] : [UI==4]
  Idle -> Bajando [order 3] : [UI==3&&S>0]
  Subiendo_hasta_arriba -> Bajand_hasta_abajo [order 3] : [UI==4]
  Idle -> Bajand_hasta_abajo [order 4] : [UI==4&&S>0]
  Bajando -> Subiendo [order 3] : [UI==1]
  Subiendo_hasta_arriba -> Bajando [order 4] : [UI==3]
  Bajand_hasta_abajo -> Subiendo [order 4] : [UI==1]
  Bajand_hasta_abajo -> Idle [order 1] : [S<=0]
  Bajand_hasta_abajo -> Subiendo_hasta_arriba [order 3] : [UI>2]
  Bajando -> Idle [order 1] : [S<=0||UI==0]
  Bajando -> Subiendo_hasta_arriba [order 4] : [UI==2]
  (default) -> Idle
  Idle -> Subiendo_hasta_arriba [order 2] : [UI==2&&S<5]
  Idle -> Subiendo [order 1] : [UI == 1&&S<5]
  Subiendo -> Idle [order 1] : [S>=5||UI==0]
  Subiendo_hasta_arriba -> Idle [order 1] : [S >=5]
  Subiendo_hasta_arriba -> Subiendo [order 2] : [UI ==1]
  Subiendo -> Subiendo_hasta_arriba [order 2] : [UI==2]
  data: S input; UI input; W output double

== stateflow chart c00026M_harness/M079/Cyber/WL1/Chart1 ==
  state Bajand_hasta_abajo
    entry: W = -1;
  state Bajando
    entry: W = -1;
  state Idle
    entry:W = 0;
  state Subiendo_hasta_arriba
    entry: W = 1;
  state Subiendo
    entry: W = 1;
  Subiendo -> Bajand_hasta_abajo [order 4] : [UI==4]
  Bajand_hasta_abajo -> Bajando [order 2] : [UI==3]
  Subiendo -> Bajando [order 3] : [UI==3]
  Bajando -> Bajand_hasta_abajo [order 2] : [UI==4]
  Idle -> Bajando [order 3] : [UI==3&&S>0]
  Subiendo_hasta_arriba -> Bajand_hasta_abajo [order 3] : [UI==4]
  Idle -> Bajand_hasta_abajo [order 4] : [UI==4&&S>0]
  Bajando -> Subiendo [order 3] : [UI==1]
  Subiendo_hasta_arriba -> Bajando [order 4] : [UI==3]
  Bajand_hasta_abajo -> Subiendo [order 4] : [UI==1]
  Bajand_hasta_abajo -> Idle [order 1] : [S<=0]
  Bajand_hasta_abajo -> Subiendo_hasta_arriba [order 3] : [UI==2]
  Bajando -> Idle [order 1] : [S<=0||UI==0]
  Bajando -> Subiendo_hasta_arriba [order 4] : [UI==2]
  (default) -> Idle
  Idle -> Subiendo_hasta_arriba [order 2] : [UI==2&&S<5]
  Idle -> Subiendo [order 1] : [UI == 1&&S<5]
  Subiendo -> Idle [order 1] : [S>=5||UI==0]
  Subiendo_hasta_arriba -> Idle [order 1] : [S >=5]
  Subiendo_hasta_arriba -> Subiendo [order 2] : [UI ==1]
  Subiendo -> Subiendo_hasta_arriba [order 2] : [UI==2]
  data: S input; UI input; W output double

== stateflow chart c00026M_harness/M079/Cyber/WL3/Chart2 ==
  state Bajand_hasta_abajo
    entry: W = -1;
  state Bajando
    entry: W = -1;
  state Idle
    entry:W = 0;
  state Subiendo_hasta_arriba
    entry: W = 1;
  state Subiendo
    entry: W = 1;
  Subiendo -> Bajand_hasta_abajo [order 4] : [UI==4]
  Bajand_hasta_abajo -> Bajando [order 2] : [UI==3]
  Subiendo -> Bajando [order 3] : [UI==3]
  Bajando -> Bajand_hasta_abajo [order 2] : [UI==4]
  Idle -> Bajando [order 3] : [UI==3&&S>PosMinW4]
  Subiendo_hasta_arriba -> Bajand_hasta_abajo [order 3] : [UI==4]
  Idle -> Bajand_hasta_abajo [order 4] : [UI==4&&S>PosMinW4]
  Bajando -> Subiendo [order 3] : [UI==1]
  Subiendo_hasta_arriba -> Bajando [order 4] : [UI==3]
  Bajand_hasta_abajo -> Subiendo [order 4] : [UI==1]
  Bajand_hasta_abajo -> Idle [order 1] : [S<=PosMinW4]
  Bajand_hasta_abajo -> Subiendo_hasta_arriba [order 3] : [UI==2]
  Bajando -> Idle [order 1] : [S<=PosMinW4||UI==0]
  Bajando -> Subiendo_hasta_arriba [order 4] : [UI==2]
  (default) -> Idle
  Idle -> Subiendo_hasta_arriba [order 2] : [UI==2&&S<5]
  Idle -> Subiendo [order 1] : [UI == 1&&S<5]
  Subiendo -> Idle [order 1] : [S>=5||UI==0]
  Subiendo_hasta_arriba -> Idle [order 1] : [S >=5]
  Subiendo_hasta_arriba -> Subiendo [order 2] : [UI ==1]
  Subiendo -> Subiendo_hasta_arriba [order 2] : [UI==2]
  data: S input; UI input; W output double; PosMinW4 input

== stateflow chart c00026M_harness/M080/Cyber/WL/Chart ==
  state Bajand_hasta_abajo
    entry: W = -1;
  state Bajando
    entry: W = -1;
  state Idle
    entry:W = 0;
  state Subiendo_hasta_arriba
    entry: W = 1;
  state Subiendo
    entry: W = 1;
  Subiendo -> Bajand_hasta_abajo [order 4] : [UI==4]
  Bajand_hasta_abajo -> Bajando [order 2] : [UI==3]
  Subiendo -> Bajando [order 3] : [UI==3]
  Bajando -> Bajand_hasta_abajo [order 2] : [UI==4]
  Idle -> Bajando [order 3] : [UI==3&&S>0]
  Subiendo_hasta_arriba -> Bajand_hasta_abajo [order 3] : [UI==4]
  Idle -> Bajand_hasta_abajo [order 4] : [UI==4&&S>0]
  Bajando -> Subiendo [order 3] : [UI==1]
  Subiendo_hasta_arriba -> Bajando [order 4] : [UI==3]
  Bajand_hasta_abajo -> Subiendo [order 4] : [UI==1]
  Bajand_hasta_abajo -> Idle [order 1] : [S<=0]
  Bajand_hasta_abajo -> Subiendo_hasta_arriba [order 3] : [UI==2]
  Bajando -> Idle [order 1] : [S<=0||UI==0]
  Bajando -> Subiendo_hasta_arriba [order 4] : [UI==2]
  (default) -> Idle
  Idle -> Subiendo_hasta_arriba [order 2] : [UI==2&&S<5]
  Idle -> Subiendo [order 1] : [UI == 1&&S<5]
  Subiendo -> Idle [order 1] : [S>=5||UI==0]
  Subiendo_hasta_arriba -> Idle [order 1] : [S >=5]
  Subiendo_hasta_arriba -> Subiendo [order 2] : [UI ==1]
  Subiendo -> Subiendo_hasta_arriba [order 2] : [UI==2]
  data: S input; UI input; W output double

== stateflow chart c00026M_harness/M080/Cyber/WL1/Chart1 ==
  state Bajand_hasta_abajo
    entry: W = -1;
  state Bajando
    entry: W = -1;
  state Idle
    entry:W = 0;
  state Subiendo_hasta_arriba
    entry: W = 1;
  state Subiendo
    entry: W = 1;
  Subiendo -> Bajand_hasta_abajo [order 4] : [UI==4]
  Bajand_hasta_abajo -> Bajando [order 2] : [UI==3]
  Subiendo -> Bajando [order 3] : [UI==3]
  Bajando -> Bajand_hasta_abajo [order 2] : [UI==4]
  Idle -> Bajando [order 3] : [UI==3&&S>0]
  Subiendo_hasta_arriba -> Bajand_hasta_abajo [order 3] : [UI==4]
  Idle -> Bajand_hasta_abajo [order 4] : [UI==4&&S>0]
  Bajando -> Subiendo [order 3] : [UI==1]
  Subiendo_hasta_arriba -> Bajando [order 4] : [UI==3]
  Bajand_hasta_abajo -> Subiendo [order 4] : [UI==1]
  Bajand_hasta_abajo -> Idle [order 1] : [S<=0]
  Bajand_hasta_abajo -> Subiendo_hasta_arriba [order 3] : [UI>2]
  Bajando -> Idle [order 1] : [S<=0||UI==0]
  Bajando -> Subiendo_hasta_arriba [order 4] : [UI==2]
  (default) -> Idle
  Idle -> Subiendo_hasta_arriba [order 2] : [UI==2&&S<5]
  Idle -> Subiendo [order 1] : [UI == 1&&S<5]
  Subiendo -> Idle [order 1] : [S>=5||UI==0]
  Subiendo_hasta_arriba -> Idle [order 1] : [S >=5]
  Subiendo_hasta_arriba -> Subiendo [order 2] : [UI ==1]
  Subiendo -> Subiendo_hasta_arriba [order 2] : [UI==2]
  data: S input; UI input; W output double

== stateflow chart c00026M_harness/M080/Cyber/WL3/Chart2 ==
  state Bajand_hasta_abajo
    entry: W = -1;
  state Bajando
    entry: W = -1;
  state Idle
    entry:W = 0;
  state Subiendo_hasta_arriba
    entry: W = 1;
  state Subiendo
    entry: W = 1;
  Subiendo -> Bajand_hasta_abajo [order 4] : [UI==4]
  Bajand_hasta_abajo -> Bajando [order 2] : [UI==3]
  Subiendo -> Bajando [order 3] : [UI==3]
  Bajando -> Bajand_hasta_abajo [order 2] : [UI==4]
  Idle -> Bajando [order 3] : [UI==3&&S>PosMinW4]
  Subiendo_hasta_arriba -> Bajand_hasta_abajo [order 3] : [UI==4]
  Idle -> Bajand_hasta_abajo [order 4] : [UI==4&&S>PosMinW4]
  Bajando -> Subiendo [order 3] : [UI==1]
  Subiendo_hasta_arriba -> Bajando [order 4] : [UI==3]
  Bajand_hasta_abajo -> Subiendo [order 4] : [UI==1]
  Bajand_hasta_abajo -> Idle [order 1] : [S<=PosMinW4]
  Bajand_hasta_abajo -> Subiendo_hasta_arriba [order 3] : [UI==2]
  Bajando -> Idle [order 1] : [S<=PosMinW4||UI==0]
  Bajando -> Subiendo_hasta_arriba [order 4] : [UI==2]
  (default) -> Idle
  Idle -> Subiendo_hasta_arriba [order 2] : [UI==2&&S<5]
  Idle -> Subiendo [order 1] : [UI == 1&&S<5]
  Subiendo -> Idle [order 1] : [S>=5||UI==0]
  Subiendo_hasta_arriba -> Idle [order 1] : [S >=5]
  Subiendo_hasta_arriba -> Subiendo [order 2] : [UI ==1]
  Subiendo -> Subiendo_hasta_arriba [order 2] : [UI==2]
  data: S input; UI input; W output double; PosMinW4 input
